simulink subsystem "Logica_evitaparedes_simple"  (R2023b)
settings: Solver=VariableStepAuto  StartTime=0.0  StopTime=10.0  RelTol=1e-3
libraries: simulink x2
settings Model: Creator=34611  LastModifiedBy=34611

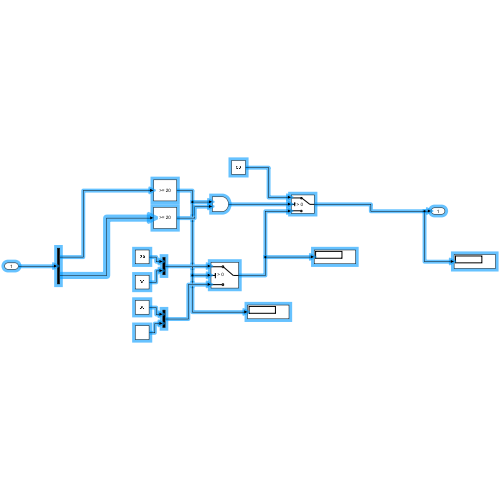
[thumbnail: Simulink's stored preview of the top-level diagram]
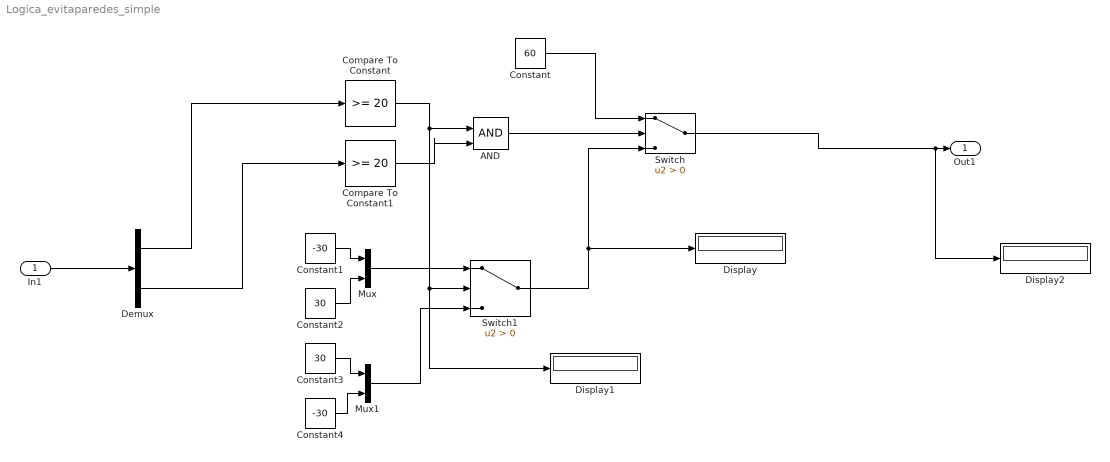
== system Logica_evitaparedes_simple ==
  In1 : Inport
  AND : Logic  IconShape=distinctive  AllPortsSameDT=off  OutDataTypeStr=boolean
  Compare To Constant : simulink/Logic and Bit Operations/Compare To Constant  relop=>=  const=20  OutDataTypeStr=uint8
  Compare To Constant1 : simulink/Logic and Bit Operations/Compare To Constant  relop=>=  const=20  OutDataTypeStr=uint8
  Constant : Constant  Value=60
  Constant1 : Constant  Value=-30
  Constant2 : Constant  Value=30
  Constant3 : Constant  Value=30
  Constant4 : Constant  Value=-30
  Demux : Demux  Outputs=2
  Display : Display
  Display1 : Display
  Display2 : Display
  Mux : Mux  Inputs=2
  Mux1 : Mux  Inputs=2
  Switch : Switch  Criteria=u2 > Threshold  SaturateOnIntegerOverflow=off  InputSameDT=off
  Switch1 : Switch  Criteria=u2 > Threshold  SaturateOnIntegerOverflow=off  InputSameDT=off
  Out1 : Outport
  wires:
  Constant1/1 -> Mux/1
  Switch1/1 -> Switch/3, Display/1
  Mux/1 -> Switch1/1
  Compare To Constant1/1 -> AND/2
  Constant4/1 -> Mux1/2
  Mux1/1 -> Switch1/3
  Constant/1 -> Switch/1
  Switch/1 -> Display2/1, Out1/1
  Constant3/1 -> Mux1/1
  Compare To Constant/1 -> Display1/1, Switch1/2, AND/1
  In1/1 -> Demux/1
  Constant2/1 -> Mux/2
  Demux/1 -> Compare To Constant/1
  AND/1 -> Switch/2
  Demux/2 -> Compare To Constant1/1
